simulink model "Anillos_Sim"  (Simulink 9.3)
settings: Solver=ode45  StartTime=0.0  StopTime=20.0  RelTol=1e-3  EnableMultiTasking=on
values from neighbouring files (symbols this model uses):
  De = conv(Se,N)    [T_Anillos.m]
  gg = num(2)/den(6)    [T_Anillos.m]
  M = conv([1 1],[1 1 1])    [T_Anillos.m]
  N = [2 2*a]    [T_Anillos.m]
  Rd = [coef(4) coef(5) coef(6)]    [T_Anillos.m]
  Sd = [coef(1) coef(2) coef(3)]    [T_Anillos.m]
undefined symbols (not defined in the file or in its folder): Re
settings Model: Creator=Tlayekanketl  LastModifiedBy=Tlakatl
settings DataIOCC: LimitDataPoints=on  SignalLoggingSaveFormat=Dataset
settings DebuggingCC: FcnCallInpInsideContextMsg=error  AllowSymbolicDim=off  StateNameClashWarn=warning
settings GRTTargetCC: GeneratePreprocessorConditionals=Disable all  CombineOutputUpdateFcns=on  GRTInterface=off
settings ConfigComp: CovSFcnEnable=off

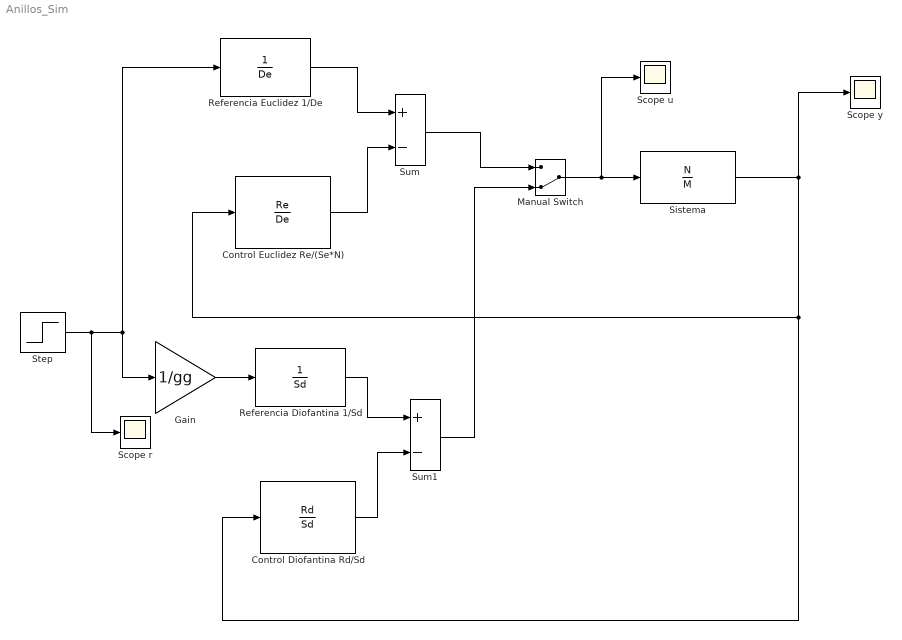
== system Anillos_Sim ==
  Control Diofantina Rd/Sd : TransferFcn  Numerator=Rd  Denominator=Sd
  Control Euclidez Re/(Se*N) : TransferFcn  Numerator=Re  Denominator=De
  Gain : Gain  Gain=1/gg
  Manual Switch : ManualSwitch  CurrentSetting=0
  Referencia Diofantina 1/Sd : TransferFcn  Denominator=Sd
  Referencia Euclidez 1/De : TransferFcn  Denominator=De
  Scope r : Scope
  Scope u : Scope
  Scope y : Scope
  Sistema : TransferFcn  Numerator=N  Denominator=M
  Step : Step  SampleTime=0
  Sum : Sum  Inputs=+-
  Sum1 : Sum  Inputs=+-
  wires:
  Step/1 -> Scope r/1, Gain/1, Referencia Euclidez 1/De/1
  Sistema/1 -> Control Diofantina Rd/Sd/1, Control Euclidez Re/(Se*N)/1, Scope y/1
  Referencia Euclidez 1/De/1 -> Sum/1
  Control Euclidez Re/(Se*N)/1 -> Sum/2
  Manual Switch/1 -> Scope u/1, Sistema/1
  Sum/1 -> Manual Switch/1
  Referencia Diofantina 1/Sd/1 -> Sum1/1
  Control Diofantina Rd/Sd/1 -> Sum1/2
  Sum1/1 -> Manual Switch/2
  Gain/1 -> Referencia Diofantina 1/Sd/1
